simulink model "MSFartoystyring2"  (R2015b)
settings: Solver=ode45  StartTime=tstart  StopTime=tstop  RelTol=1e-3
values from neighbouring files (symbols this model uses):
  c = 0    [matlab.mat]    (also in run.m; run_2_3.m = 1; test.m)
  Kd_heading = 2 * zeta_h*T-1    (= 373)    [test.m]
  Ki_heading = wn_h/10 *Kp_heading    (= 0.140312434807)    [test.m]
  Ki_speed = 1    [run.m]    (also in test.m = 0)
  Kp_heading = (T/K *wn_h^2)    (= 20.4417882877)    [test.m]
  Kp_speed = 10    [run.m]    (also in test.m = 2)
  psi0 = 0    [matlab.mat]    (also in run.m; run_2_3.m; test.m)
  r0 = 0    [matlab.mat]    (also in run.m; run_2_3.m; test.m)
  tsamp = 10    [matlab.mat]    (also in run.m; run_2_3.m; test.m)
  v0 = [6.63 0]    [matlab.mat]    (also in run.m = [6.63 0]'; run_2_3.m = [6.63 0]'; test.m = [6.63 0]')
  WP = [-600  4680  7662  10644  13626; 0  3880  2248  3878  2246]    [matlab.mat]
undefined symbols (not defined in the file or in its folder): delta_c, delta_offset, msfartoystyring
undefined symbols (not defined in the file): p0
libraries: simulink_extras x1
settings Model: ExtModeAutoUpdateStatusClock=off  Creator=christh  LastModifiedBy=ShivJeet
settings DataIOCC: SaveFormat=Array  SignalLoggingSaveFormat=ModelDataLogs
settings OptimizationCC: ExpressionDepthLimit=2147483647  InitFltsAndDblsToZero=on
settings DebuggingCC: UnderspecifiedInitializationDetection=Classic  MergeDetectMultiDrivingBlocksExec=none  SolverPrmCheckMsg=warning  FcnCallInpInsideContextMsg=UseLocalSettings  StateNameClashWarn=warning
settings HardwareCC: ProdBitPerPointer=32  ProdLargestAtomicFloat=None  ProdIntDivRoundTo=Undefined  ProdEndianess=Unspecified  ProdWordSize=32  ProdHWDeviceType=32-bit Generic
settings GRTTargetCC: GeneratePreprocessorConditionals=Disable all  CombineOutputUpdateFcns=off  GRTInterface=on
settings ConfigComp: CovModelRefEnable=Off

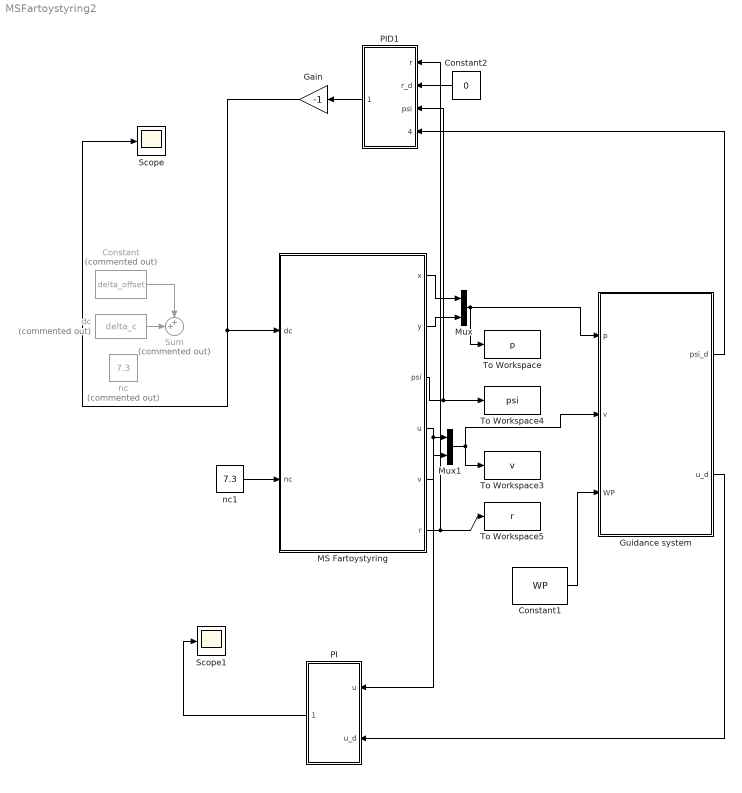
== system MSFartoystyring2 ==
  Constant : Constant  Commented=on  Value=delta_offset
  Constant1 : Constant  Value=WP
  Constant2 : Constant  Value=0
  Gain : Gain  Gain=-1
  Guidance system : Subsystem
  MS Fartoystyring : Subsystem  mask(MS Fartoystyring for Assignment 3 G&C){x0=p0(1), y0=p0(2), u0=v0(1), v0=v0(2), psi0=psi0, r0=r0, c=c}
      mask prompts: x0 "x(t0) (m)"; y0 "y(t0) (m)"; u0 "u(t0) (m/s)"; v0 "v(t0) (m/s)"; psi0 "psi(t0) (rad)"; r0 "r(t0) (rad/s)"; c "current (0 or 1)"
      mask help:
      | Block corresponding to Figure 1 in the assignment text. Gives the response of the ship.
      |
      | The design speed of MS Fartoystyring is u=8.23 m/s.
      |
      | Input:
      | dc: commanded rudder (rad), dmax=25*pi/180
      | nc: commanded shaft speed (rad/s), nmax=85*2*pi/60
      |
      | Output:
      | x: north pos (m)
      | y: east pos (m)
      | u: surge (m/s)
      | v: sway (m/s)
      | psi: heading (rad)
      | r: yaw (rad/s)
      mask Help: Comments, bugs and help requests can be directed to the TA. Email on course website.
  Mux : Mux  Inputs=2
  Mux1 : Mux  Inputs=2
  PI : Subsystem
  PID1 : Subsystem
  Scope : Scope
  Scope1 : Scope
  Sum : Sum  Commented=on  Inputs=++|
  To Workspace : ToWorkspace  VariableName=p  SampleTime=tsamp
  To Workspace3 : ToWorkspace  VariableName=v  SampleTime=tsamp
  To Workspace4 : ToWorkspace  VariableName=psi  SampleTime=tsamp
  To Workspace5 : ToWorkspace  VariableName=r  SampleTime=tsamp
  dc : Constant  Commented=on  Value=delta_c
  nc : Constant  Commented=on  Value=7.3
  nc1 : Constant  Value=7.3
  wires:
  MS Fartoystyring/1(x) -> Mux/1
  MS Fartoystyring/2(y) -> Mux/2
  MS Fartoystyring/4(u) -> PI/1(u), Mux1/1
  MS Fartoystyring/5(v) -> Mux1/2
  Mux/1 -> To Workspace/1, Guidance system/1(p)
  MS Fartoystyring/3(psi) -> PID1/3(psi), To Workspace4/1
  dc/1 -> Sum/2
  Constant/1 -> Sum/1
  Mux1/1 -> To Workspace3/1, Guidance system/2(v)
  Constant1/1 -> Guidance system/3(WP)
  Guidance system/1(psi_d) -> PID1/4(psi_d)
  Guidance system/2(u_d) -> PI/2(u_d)
  Constant2/1 -> PID1/2(r_d)
  MS Fartoystyring/6(r) -> To Workspace5/1, PID1/1(r)
  PID1/1("delta_d ") -> Gain/1
  Gain/1 -> Scope/1, MS Fartoystyring/1(dc)
  nc1/1 -> MS Fartoystyring/2(nc)
  PI/1("delta_d ") -> Scope1/1

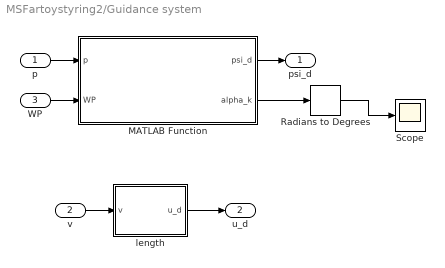
== system MSFartoystyring2/Guidance system ==
  p : Inport
  v : Inport  Port=2
  WP : Inport  Port=3
  MATLAB Function : MATLAB Function  TreatAsAtomicUnit=on
  Radians to Degrees : simulink_extras/Transformations/Radians to Degrees
  Scope : Scope
  length : MATLAB Function  TreatAsAtomicUnit=on
  psi_d : Outport
  u_d : Outport  Port=2
  wires:
  p/1 -> MATLAB Function/1(p)
  v/1 -> length/1(v)
  length/1(u_d) -> u_d/1
  WP/1 -> MATLAB Function/2(WP)
  MATLAB Function/1(psi_d) -> psi_d/1
  MATLAB Function/2(alpha_k) -> Radians to Degrees/1
  Radians to Degrees/1 -> Scope/1

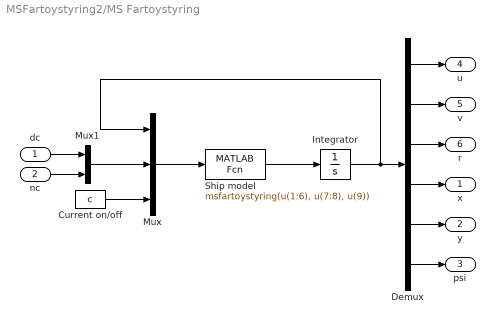
== system MSFartoystyring2/MS Fartoystyring ==
  dc : Inport
  nc : Inport  Port=2
  Current on/off : Constant  Value=c
  Demux : Demux  Outputs=6
  Integrator : Integrator  InitialCondition=[u0 v0 r0 x0 y0 psi0]'
  Mux : Mux  Inputs=3
  Mux1 : Mux  Inputs=2
  Ship model : MATLABFcn  MATLABFcn=msfartoystyring(u(1:6), u(7:8), u(9))  OutputDimensions=6
  x : Outport
  y : Outport  Port=2
  psi : Outport  Port=3
  u : Outport  Port=4
  v : Outport  Port=5
  r : Outport  Port=6
  wires:
  Integrator/1 -> Mux/1, Demux/1
  dc/1 -> Mux1/1
  nc/1 -> Mux1/2
  Demux/1 -> u/1
  Demux/2 -> v/1
  Demux/3 -> r/1
  Demux/4 -> x/1
  Demux/5 -> y/1
  Demux/6 -> psi/1
  Current on/off/1 -> Mux/3
  Ship model/1 -> Integrator/1
  Mux/1 -> Ship model/1
  Mux1/1 -> Mux/2

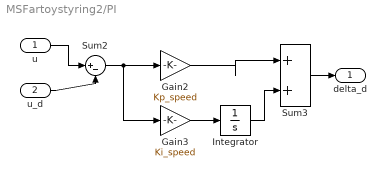
== system MSFartoystyring2/PI ==
  u : Inport
  u_d : Inport  Port=2
  Gain2 : Gain  Gain=Kp_speed
  Gain3 : Gain  Gain=Ki_speed
  Integrator : Integrator
  Sum2 : Sum  Inputs=|+-
  Sum3 : Sum  Inputs=|++
  "delta_d " : Outport
  wires:
  Sum3/1 -> "delta_d "/1
  u/1 -> Sum2/1
  u_d/1 -> Sum2/2
  Sum2/1 -> Gain2/1, Gain3/1
  Gain3/1 -> Integrator/1
  Gain2/1 -> Sum3/1
  Integrator/1 -> Sum3/2

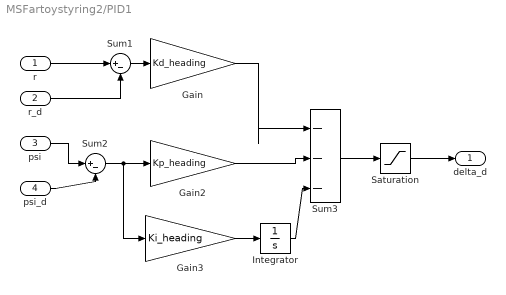
== system MSFartoystyring2/PID1 ==
  r : Inport
  r_d : Inport  Port=2
  psi : Inport  Port=3
  psi_d : Inport  Port=4
  Gain : Gain  Gain=Kd_heading
  Gain2 : Gain  Gain=Kp_heading
  Gain3 : Gain  Gain=Ki_heading
  Integrator : Integrator
  Saturation : Saturate  UpperLimit=deg2rad(25)  LowerLimit=-deg2rad(25)
  Sum1 : Sum  Inputs=|+-
  Sum2 : Sum  Inputs=|+-
  Sum3 : Sum  Inputs=|---
  "delta_d " : Outport
  wires:
  r/1 -> Sum1/1
  r_d/1 -> Sum1/2
  Sum1/1 -> Gain/1
  psi/1 -> Sum2/1
  psi_d/1 -> Sum2/2
  Sum2/1 -> Gain2/1, Gain3/1
  Gain2/1 -> Sum3/2
  Gain3/1 -> Integrator/1
  Integrator/1 -> Sum3/3
  Gain/1 -> Sum3/1
  Sum3/1 -> Saturation/1
  Saturation/1 -> "delta_d "/1

== matlab function MSFartoystyring2/Guidance system/length ==
  data: v input; u_d output
function u_d = fcn(v)
%#codegen
u_d = sqrt(v(1)^2 +v(2)^2);
end

== matlab function MSFartoystyring2/Guidance system/MATLAB Function ==
  data: p input; psi_d output; WP input; alpha_k output
function [psi_d,alpha_k]  = fcn(p,WP)
persistent index

% Setting the index first time
if isempty(index)
    index = 2;
end
% Circle radius R --> length of LOS 
R = (WP(1,index) + p(1))^2 + (WP(2,index) + p(2))^2;

% Waypoint reached, moving to next waypoint
if (WP(1,index) < p(1) && WP(2,index) < p(2) && index < length(WP))
    disp('index')
    index = index + 1;
end

%% Minimizing the error (error is the difference between ship and the desired path)
y_LOS = 0;
x_LOS = 0;
dy = WP(2,index) - WP(2,index-1);
dx = WP(1,index) - WP(1,index-1);
alpha_k = atan2(dy,dx);
%Checking how far the next waypoint is from the previous 
if (abs(dx) > 0)

    d = dy/dx;
    e = WP(1,index-1);
    f = WP(2,index-1);
    g = f-d*e;

    a = 1 + d^2;
    b = 2*(d*g -d*p(2) - p(1));
    c = p(1)^2 + p(2)^2 + g^2 - 2*g*p(2) - R^2;
    disp('b^2-4*a*c')
    disp(b^2-4*a*c)
    
    if (dx >0)
        x_LOS =(-b+sqrt(b^2-4*a*c))/(2*a);
    else
        x_LOS = (-b-sqrt(b^2-4*a*c))/(2*a);
    end
else
    x_LOS = WP(1,index-1); % or WP(1,index); X-value is the same
end
disp('R^2 -(x_LOS - p(1))')
disp(R^2 -(x_LOS - p(1)))
if abs(dy) > 0
    if dy > 0
        y_LOS = p(2) + sqrt(R^2 -(x_LOS - p(1))^2);
    else
        y_LOS = p(2) - sqrt(R^2 -(x_LOS - p(1))^2);
    end
else 
    y_LOS = WP(2,index-1); % or WP(2,index+1); Y-value is the same
end

psi_d = atan2(y_LOS - p(2),x_LOS-p(1));                                      % angle between the desired waypoint and the current position of the ship
end
